simulink model "FlexAxleSpeedgoatBaseline"  (R2025b)
settings: Solver=FixedStepDiscrete  StartTime=0.0  StopTime=inf  FixedStep=0.001  RelTol=1e-3
undefined symbols (not defined in the file): IO397, Pull, pull, Ts, up
libraries: speedgoatlib_fpga_analog_io x3, speedgoatlib_fpga_quadrature x3, speedgoatlib_fpga_dio x1, speedgoatlib_fpga_inta x1, simulink x1, speedgoatlib_interrupt x1, speedgoatlib_fpga_pwm x1, speedgoatlib_fpga x1
settings Model: SimulationMode=external  ExtModeEnableFloating=off  Creator=jeffrey.gruenig  LastModifiedBy=gertv
settings SolverCC: ConcurrentTasks=on  PositivePriorityOrder=on
settings DataIOCC: SaveFormat=StructureWithTime
settings OptimizationCC: BlockReduction=off  OptimizeBlockIOStorage=off  BufferReuse=off
settings DebuggingCC: UnderspecifiedInitializationDetection=Classic  MergeDetectMultiDrivingBlocksExec=none  TasksWithSamePriorityMsg=none
settings HardwareCC: ProdBitPerLong=64.0  ProdLongLongMode=on  ProdHWDeviceType=Intel->x86-64 (Linux 64)
settings ModelReferenceCC: PropagateSignalLabelsOutOfModel=off
settings RTWCC: SystemTargetFile=speedgoat.tlc  TemplateMakefile=slrealtime_default_tmf  Toolchain=Simulink Real-Time Toolchain  BuildConfiguration=Faster Runs  CodeExecutionProfiling=on  TargetLang=C++  Description=Speedgoat Real-Time Target Machine
settings SimulinkRealTimeTargetCC: SLRTFileLogMaxRuns=1.0  ExtModeMaxTrigDuration=10.0  ExtModeStaticAllocSize=1000000.0  ExtModeTransport=0.0  MultiwordLength=2048.0  DynamicStringBufferSize=256.0  PreserveMATLABNamespacesInGeneratedCode=on  SubcomponentCodeInterfacePackaging=Reusable function  InstructionSetFMA=off  LogToMDFFile=off

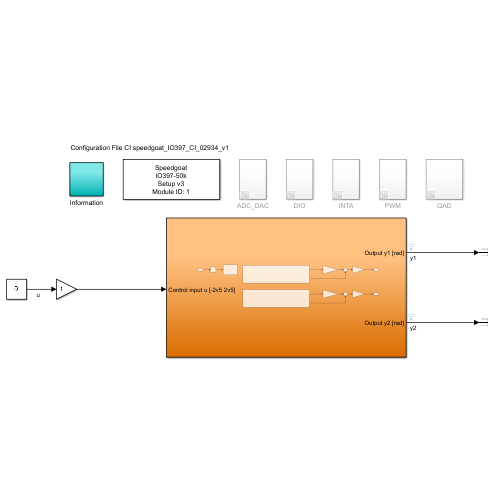
[thumbnail: Simulink's stored preview of the top-level diagram]
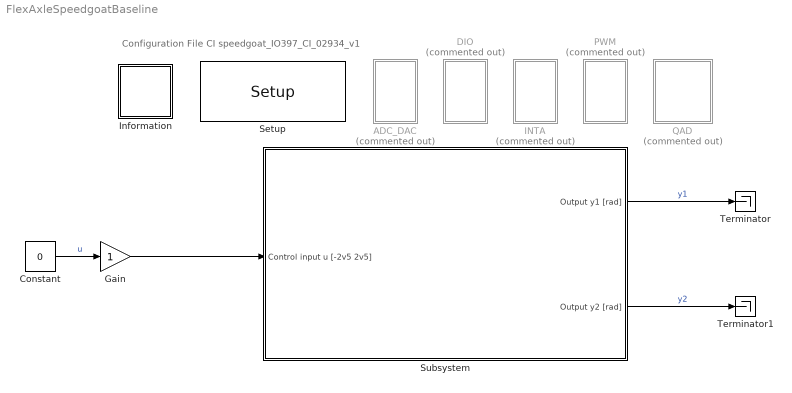
== system FlexAxleSpeedgoatBaseline ==
  note: Configuration File CI speedgoat_IO397_CI_02934_v1
  ADC_DAC : Subsystem  Commented=on
  Constant : Constant  Value=0
  DIO : Subsystem  Commented=on
  Gain : Gain
  INTA : Subsystem  Commented=on
  Information : Subsystem
  PWM : Subsystem  Commented=on
  QAD : Subsystem  Commented=on
  Setup : speedgoatlib_fpga/Setup/Setup  board=IO397-50k  id=1  pciSlot=-1  device_id=1  bitstreamFilePath=C:\Users\gertv\Documents\Werk\Continuing Thesis\Matlab\GithubFolder\Section 9 - Experimental Results\ExperimentSet_up\DeePC_Exp  bitstreamFile=speedgoat_IO397_CI_02934_v1.mat  fpgaFreq=75000000  enableDma=off  rearEnb_1=off  rearIO_1=None  rearEnb_2=off  rearIO_2=None  ProgSpiFlash=off  ProgBPIFlash=off  useFpgaDmaController=off  dmaStopOnOverload=on  dmaModeSequential=on  dmaModeParallel=off  dmaTrigFixTime=on  dmaTrigA2B=off  dmaTriggerSourceSel=0  PullRPort15=pull-up 3.3V  PullRPort31=pull-up 3.3V  PullRPort47=pull-up 3.3V  PullRPort63=pull-up 3.3V  diffLineTermination_1=on  diffLineTermination_2=on  diffLineTermination_3=on  diffLineTermination_4=on  diffLineTermination_5=on  diffLineTermination_6=on  diffLineTermination_7=on  diffLineTermination_8=on  diffLineTermination_9=on  diffLineTermination_10=on  diffLineTermination_11=on  diffLineTermination_12=on  diffLineTermination_13=on  diffLineTermination_14=on  diffLineTermination_15=on  diffLineTermination_16=on  diffLineTermination_17=on  diffLineTermination_18=on  diffLineTermination_19=on  diffLineTermination_20=on  diffLineTermination_21=on  diffLineTermination_22=on  diffLineTermination_23=on  diffLineTermination_24=on  diffLineTermination_25=on  diffLineTermination_26=on  diffLineTermination_27=on  diffLineTermination_28=on  diffLineTermination_29=on  diffLineTermination_30=on  diffLineTermination_31=on  diffLineTermination_32=on  ioVoltageDropDown1=3.3V  pullResistorDropDown1_1=Pull-up  pullResistorDropDown1_2=Pull-up  pullResistorDropDown1_3=Pull-up  pullResistorDropDown1_4=Pull-up  pullResistorDropDown1_5=Pull-up  pullResistorDropDown1_6=Pull-up  pullResistorDropDown1_7=Pull-up  pullResistorDropDown1_8=Pull-up  ttlIsImplementedCheckBox1=off  pullResistorDropDown2=Pull-up  ioVoltageDropDown2=3.3V  ttlIsImplementedCheckBox2=off  pullResistorDropDown3=Pull-up  ioVoltageDropDown3=3.3V  ttlIsImplementedCheckBox3=off  pullResistorDropDown4=Pull-up  ioVoltageDropDown4=3.3V  ttlIsImplementedCheckBox4=off  pullResistorDropDown5=Pull-up  ioVoltageDropDown5=3.3V  ttlIsImplementedCheckBox5=off  pullResistorDropDown6=Pull-up  ioVoltageDropDown6=3.3V  ttlIsImplementedCheckBox6=off  pullResistorDropDown7=Pull-up  ioVoltageDropDown7=3.3V  ttlIsImplementedCheckBox7=off  pullResistorDropDown8=Pull-up  ioVoltageDropDown8=3.3V  ttlIsImplementedCheckBox8=off  terminationCheckBox1=off  terminationCheckBox2=off  terminationCheckBox3=off  terminationCheckBox4=off  diffIsImplementedCheckBox1=off  terminationCheckBox5=off  terminationCheckBox6=off  terminationCheckBox7=off  terminationCheckBox8=off  diffIsImplementedCheckBox2=off  terminationCheckBox9=off  terminationCheckBox10=off  terminationCheckBox11=off  terminationCheckBox12=off  diffIsImplementedCheckBox3=off  terminationCheckBox13=off  terminationCheckBox14=off  terminationCheckBox15=off  terminationCheckBox16=off  diffIsImplementedCheckBox4=off  terminationCheckBox17=off  terminationCheckBox18=off  terminationCheckBox19=off  terminationCheckBox20=off  diffIsImplementedCheckBox5=off  terminationCheckBox21=off  terminationCheckBox22=off  terminationCheckBox23=off  terminationCheckBox24=off  diffIsImplementedCheckBox6=off  terminationCheckBox25=off  terminationCheckBox26=off  terminationCheckBox27=off  terminationCheckBox28=off  diffIsImplementedCheckBox7=off  terminationCheckBox29=off  terminationCheckBox30=off  terminationCheckBox31=off  terminationCheckBox32=off  diffIsImplementedCheckBox8=off  PullRPort0_1=pull-up  VioPort0_1=3.3V  PullRPort1_1=pull-up  VioPort1_1=3.3V  PullRPort2_1=pull-up  VioPort2_1=3.3V  PullRPort3_1=pull-up  VioPort3_1=3.3V  PullRPort4_1=pull-up  VioPort4_1=3.3V  PullRPort5_1=pull-up  VioPort5_1=3.3V  PullRPort6_1=pull-up  VioPort6_1=3.3V  diffLineTermination_rear1_1=on  diffLineTermination_rear1_2=on  diffLineTermination_rear1_3=on  diffLineTermination_rear1_4=on  diffLineTermination_rear1_5=on  diffLineTermination_rear1_6=on  diffLineTermination_rear1_7=on  diffLineTermination_rear1_8=on  PullRPort0_2=pull-up  VioPort0_2=3.3V  PullRPort1_2=pull-up  VioPort1_2=3.3V  PullRPort2_2=pull-up  VioPort2_2=3.3V  PullRPort3_2=pull-up  VioPort3_2=3.3V  PullRPort4_2=pull-up  VioPort4_2=3.3V  PullRPort5_2=pull-up  VioPort5_2=3.3V  PullRPort6_2=pull-up  VioPort6_2=3.3V  diffLineTermination_rear2_1=on  diffLineTermination_rear2_2=on  diffLineTermination_rear2_3=on  diffLineTermination_rear2_4=on  diffLineTermination_rear2_5=on  diffLineTermination_rear2_6=on  diffLineTermination_rear2_7=on  diffLineTermination_rear2_8=on
      settings: SourceProductName=IO3xx
  Subsystem : Subsystem
  Terminator : Terminator
  Terminator1 : Terminator
  wires:
  Subsystem/1(Output y1 [rad]) -> Terminator/1  "y1"
  Subsystem/2(Output y2 [rad]) -> Terminator1/1  "y2"
  Constant/1 -> Gain/1  "u"
  Gain/1 -> Subsystem/1(Control input u [-2v5 2v5])

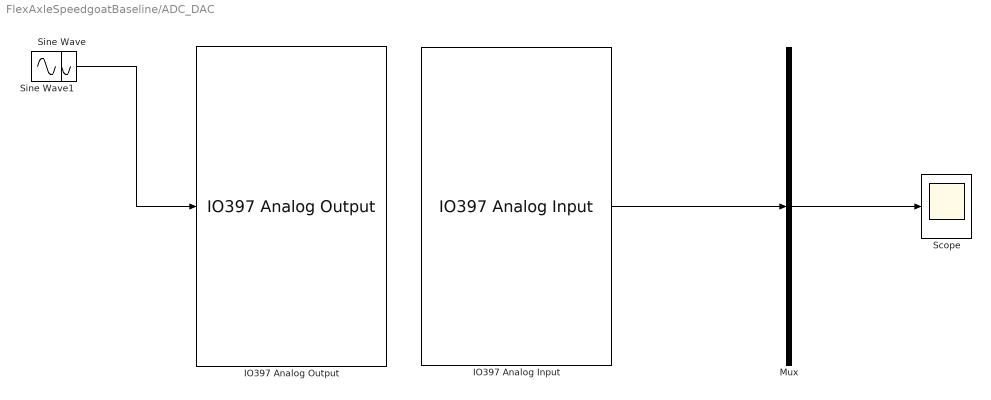
== system FlexAxleSpeedgoatBaseline/ADC_DAC ==
  IO397 Analog Input : speedgoatlib_fpga_analog_io/IO397/IO397 Analog Input  openMaskCallback=0  id=1  chan=1,  range=+5.12 V  parAiTriggerMode=I/O Module Clock  parAiInternalSignal=None  parAiDioTriggerChannel=1  parAiSampleRate=0  trigger=Initiator  ts=Ts*0.1
      settings: SourceProductName=Analog IO
  IO397 Analog Output : speedgoatlib_fpga_analog_io/IO397/IO397 Analog Output  id=1  chan=1,  initVal=0  resetVal=0  ts=0.001  span=+-10 V
      settings: SourceProductName=Analog IO
  Mux : Mux  Inputs=1
  Scope : Scope
  Sine Wave : Sin  Frequency=2*pi*(1/Ts)/50  SampleTime=Ts
  Sine Wave1 : Sin  Frequency=2*pi*(1/Ts)/50  SampleTime=Ts
  wires:
  Mux/1 -> Scope/1
  IO397 Analog Input/1 -> Mux/1
  Sine Wave/1 -> IO397 Analog Output/1

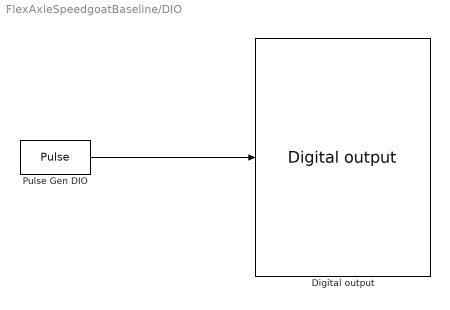
== system FlexAxleSpeedgoatBaseline/DIO ==
  Digital output : speedgoatlib_fpga_dio/Digital output  id=1  chan=[11:13]  init=[0]  reset=[0]  ts=Ts  vectorizeInput=on
      settings: SourceProductName=Digital
  Pulse Gen DIO : DiscretePulseGenerator  Period=20  PulseWidth=10  PhaseDelay=[0:5:10]  SampleTime=Ts  VectorParams1D=off
  wires:
  Pulse Gen DIO/1 -> Digital output/1

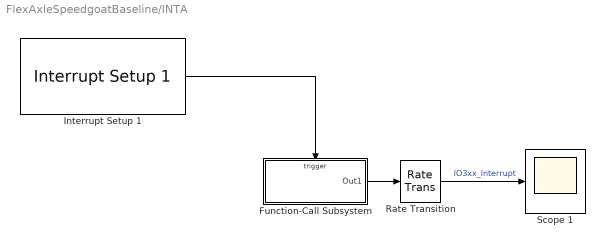
== system FlexAxleSpeedgoatBaseline/INTA ==
  Function-Call Subsystem : Subsystem  TreatAsAtomicUnit=on
  Interrupt Setup 1 : speedgoatlib_interrupt/Interrupt Setup 1  parModuleTrigger=off  parPollingMode=off  parPriorityConf=High  parPriority=241  confStartFcn=''  confStopFcn=''  confIsrFcn=''  confMapFcn=''  confHookFile=''  confIrqNr='-1'  confIsPolling=off  confModID='1'  confSelectedInt=Speedgoat IO397-50k interrupt  confSelectedId=1  confSelectedChannel=[]
  Rate Transition : RateTransition  Integrity=off
  "Scope 1 " : Scope
  wires:
  Rate Transition/1 -> "Scope 1 "/1  "IO3xx_Interrupt"
  Function-Call Subsystem/1(Out1) -> Rate Transition/1
  Interrupt Setup 1/1 -> Function-Call Subsystem/Trigger

== system FlexAxleSpeedgoatBaseline/Information ==
  note: Front I/O (Analog):
      | From Pin To Pin Tested Functionality
      | 9 1 / 2 DAC channel 1 to ADC channel 1
      | Front I/O:
      | From Pin To Pin Tested Functionality
      | 3b 12b PWM - A channel 1 to INTA channel 1
      | 13b 6b DIO channel 11 to QAD - A channel 1
      | 14b 7b DIO channel 12 to QAD - B channel 1
      | 15b 8b DIO channel 13 to QAD - C_Index channel 1

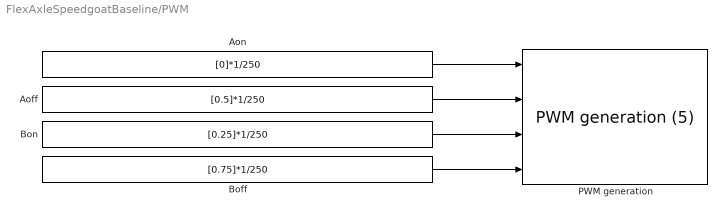
== system FlexAxleSpeedgoatBaseline/PWM ==
  Aoff : Constant  Value=[0.5]*1/250  OutDataTypeStr=Inherit: Inherit via back propagation  SampleTime=-1
  Aon : Constant  Value=[0]*1/250  VectorParams1D=off  OutDataTypeStr=Inherit: Inherit via back propagation  SampleTime=-1
  Boff : Constant  Value=[0.75]*1/250  OutDataTypeStr=Inherit: Inherit via back propagation  SampleTime=-1
  Bon : Constant  Value=[0.25]*1/250  OutDataTypeStr=Inherit: Inherit via back propagation  SampleTime=-1
  PWM generation : speedgoatlib_fpga_pwm/PWM generation (5)  id=1  chan=[1]  board=Please select...  ts=0.001  enableDma=off  pciSlot=-1  delay=0  symmetric=Asymmetric - On and Off are freely configurable  b_is_complement_of_a=Independent of PWM A output  deadband=[0.0]  period=[1/250]  frequency=250  ticks=299999  a_on=0  a_off=0.5e-3  pwm_a_dc=[0.0]  b_on=0.25e-3  b_off=0.75e-3  pwm_b_dc=[0]  c_on=[0.0]  c_off=[0.0]  protection=Disabled: A and B can be high at the same moment  enable_latch_half_period=off  pwm_update=At period starts  bit_width_pwm_gen=24  trigger_duration=[100e-6]  trigger_period_start=on  trigger_half_of_the_period=off  trigger_a_on=off  trigger_a_off=off  trigger_b_on=off  trigger_b_off=off  show_a_input=on  show_b_input=on  show_c_input=off  show_period_input=off  show_force_stop_input=off  idle_a=Low when PWM generation is halted  idle_b=Low when PWM generation is halted  idle_c=Low when PWM generation is halted  cancels_pwm_generation=on  invert_a=off  invert_b=off  invert_c=off
      settings: SourceProductName=PWM
  wires:
  Boff/1 -> PWM generation/4
  Bon/1 -> PWM generation/3
  Aoff/1 -> PWM generation/2
  Aon/1 -> PWM generation/1

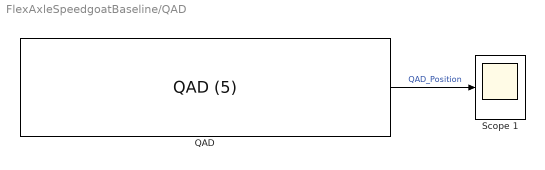
== system FlexAxleSpeedgoatBaseline/QAD ==
  QAD : speedgoatlib_fpga_quadrature/QAD (5)  id=1  chan=[1]  sampleTime=0.001  enableDma=on  numOfSlots=[16]  sensorType=Capture A + B Signal  interpolatePosition=off  swapAB=off  indexControlMode=Ignore Index  latchMode=Disabled  gateIndex=No Gating  speedFilterWidth=4  showInputSpeedFilterWidth=off  glitchFilterSeconds=106.7e-9  glitchFilterSecondsEff=106.7e-9  showInputClearPosition=off  showInputClearIndexFound=off  showOutputPosition=on  showOutputTurn=off  showOutputSpeed=off  showOutputIndexFound=off  showOutputLastPulse=off
      settings: SourceProductName=Quadrature
  "Scope 1 " : Scope
  wires:
  QAD/1 -> "Scope 1 "/1  "QAD_Position"

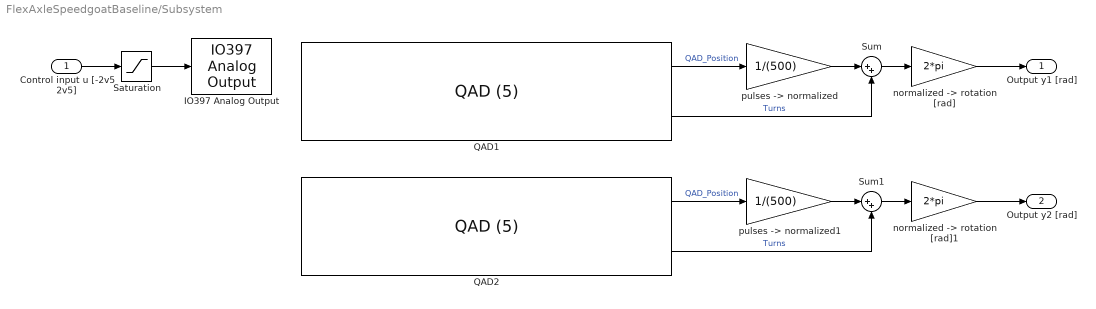
== system FlexAxleSpeedgoatBaseline/Subsystem ==
  Control input u [-2v5 2v5] : Inport
  IO397 Analog Output : speedgoatlib_fpga_analog_io/IO397/IO397 Analog Output  id=1  chan=1,  initVal=0  resetVal=1  ts=0.001  span=+-5 V
      settings: SourceProductName=Analog IO
  QAD1 : speedgoatlib_fpga_quadrature/QAD (5)  id=1  chan=[1]  sampleTime=0.001  numOfSlots=500  sensorType=Capture A + B Signal  interpolatePosition=off  swapAB=off  indexControlMode=Ignore Index  latchMode=Disabled  gateIndex=No Gating  speedFilterWidth=1  showInputSpeedFilterWidth=off  glitchFilterSeconds=0  glitchFilterSecondsEff=0  showInputClearPosition=off  showInputClearIndexFound=off  showOutputPosition=on  showOutputTurn=on  showOutputSpeed=off  showOutputIndexFound=off  showOutputLastPulse=off
      settings: SourceProductName=Quadrature
  QAD2 : speedgoatlib_fpga_quadrature/QAD (5)  id=1  chan=[2]  sampleTime=0.001  numOfSlots=500  sensorType=Capture A + B Signal  interpolatePosition=off  swapAB=off  indexControlMode=Ignore Index  latchMode=Disabled  gateIndex=No Gating  speedFilterWidth=1  showInputSpeedFilterWidth=off  glitchFilterSeconds=0  glitchFilterSecondsEff=0  showInputClearPosition=off  showInputClearIndexFound=off  showOutputPosition=on  showOutputTurn=on  showOutputSpeed=off  showOutputIndexFound=off  showOutputLastPulse=off
      settings: SourceProductName=Quadrature
  Saturation : Saturate  UpperLimit=2.5  LowerLimit=-2.5
  Sum : Sum  Inputs=|++
  Sum1 : Sum  Inputs=|++
  "normalized -> rotation [rad]" : Gain  Gain=2*pi
  "normalized -> rotation [rad]1" : Gain  Gain=2*pi
  "pulses -> normalized" : Gain  Gain=1/(500)
  "pulses -> normalized1" : Gain  Gain=1/(500)
  Output y1 [rad] : Outport
  Output y2 [rad] : Outport  Port=2
  wires:
  Saturation/1 -> IO397 Analog Output/1
  Sum/1 -> "normalized -> rotation [rad]"/1
  "normalized -> rotation [rad]"/1 -> Output y1 [rad]/1
  QAD1/1 -> "pulses -> normalized"/1  "QAD_Position"
  QAD1/2 -> Sum/2  "Turns"
  "pulses -> normalized"/1 -> Sum/1
  Control input u [-2v5 2v5]/1 -> Saturation/1
  "pulses -> normalized1"/1 -> Sum1/1
  QAD2/2 -> Sum1/2  "Turns"
  QAD2/1 -> "pulses -> normalized1"/1  "QAD_Position"
  Sum1/1 -> "normalized -> rotation [rad]1"/1
  "normalized -> rotation [rad]1"/1 -> Output y2 [rad]/1

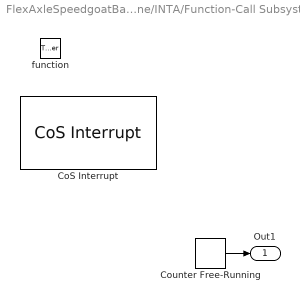
== system FlexAxleSpeedgoatBaseline/INTA/Function-Call Subsystem ==
  function : TriggerPort  TriggerType=function-call  VariantControl=Variant
  CoS Interrupt : speedgoatlib_fpga_inta/CoS Interrupt  id=1  ts=-1  debounce=0  delay=0  polarity=1
      settings: SourceProductName=Interrupt
  Counter Free-Running : simulink/Sources/Counter Free-Running  NumBits=32  tsamp=-1
  Out1 : Outport  InitialOutput=[0]  VectorParamsAs1DForOutWhenUnconnected=off
  wires:
  Counter Free-Running/1 -> Out1/1
